simulink model "SignalShapingTest"  (R2024b)
settings: Solver=VariableStepAuto  StartTime=0.0  StopTime=5  RelTol=1e-3
values from neighbouring files (symbols this model uses):
  CanaryAmplitude = 0.25    [ConfigData.sldd]
  CanaryCarrierFrequency = 20000.0    [ConfigData.sldd]
  CanaryDataRate = 100.0    [ConfigData.sldd]
  SampleRate = 48000.0    [ConfigData.sldd]
  WalshCodeIndex = 9.0 3.0    [ConfigData.sldd]
undefined symbols (not defined in the file or in its folder): magnitude
libraries: dspfdesign x5, simulink x3, commseqgen3 x3, commfilt2 x2, dspsigops x2
settings Model: DataDictionary=ConfigData.sldd  Creator=calum  LastModifiedBy=calum

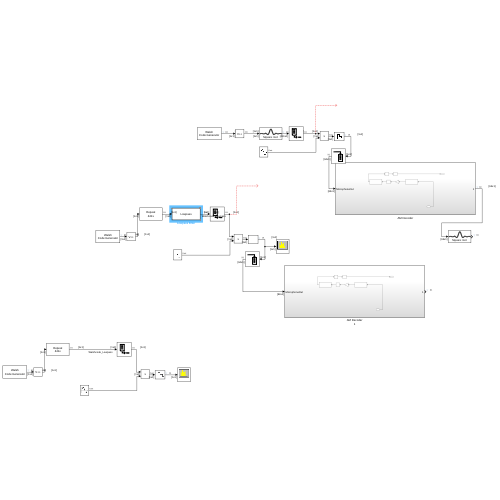
[thumbnail: Simulink's stored preview of the top-level diagram]
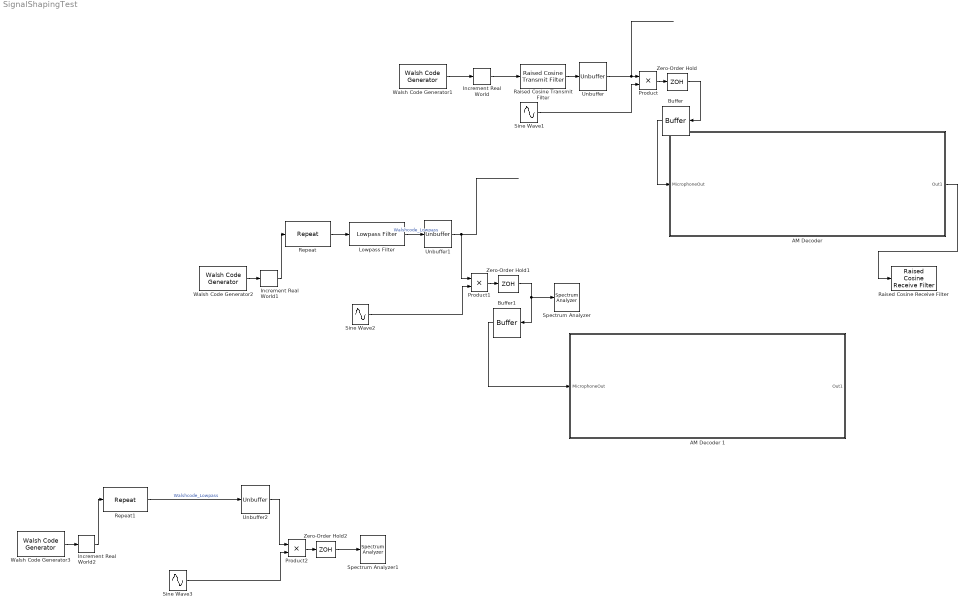
== system SignalShapingTest ==
  "AM Decoder " : Subsystem  Latency=2
  AM Decoder 1 : Subsystem  Latency=2
  Buffer : Buffer  OutputFrames=off
  Buffer1 : Buffer  OutputFrames=off
  Increment Real World : simulink/Additional Math & Discrete/Additional Math: Increment - Decrement/Increment Real World
  Increment Real World1 : simulink/Additional Math & Discrete/Additional Math: Increment - Decrement/Increment Real World
  Increment Real World2 : simulink/Additional Math & Discrete/Additional Math: Increment - Decrement/Increment Real World
  Lowpass Filter : dspfdesign/Lowpass Filter  FilterType=FIR  DesignForMinimumOrder=on  FilterOrder=50  PassbandFrequency=CanaryDataRate  StopbandFrequency=CanaryDataRate*10  PassbandRipple=0.5  StopbandAttenuation=80  SampleRateMode=Specify on dialog  SampleRate=SampleRate  SimulateUsing=Interpreted execution  roundingMode=Floor  coeffsDataTypeStr=fixdt(1,16)
  Product : Product
  Product1 : Product
  Product2 : Product
  Raised Cosine Receive Filter : commfilt2/Raised Cosine Receive Filter  filtType=Square root  R=0.2  filtSpan=2  N=SampleRate/CanaryDataRate  downFactor=1  downOffset=0  filterGain=1  InputProcessing=Columns as channels (frame based)  RateOptions=Allow multirate processing  framing=Mute  checkCoeff=off  variableName=rcRxFilt  currentFiltSpan=10  D=5  inputOffset=0  sampMode=Mute  saveAsFlag=0  rateMode=Downsampling  checkGain=Normalized  launchFVT=on  roundingMode=Floor  overflowMode=off  coeffDataTypeStr=Inherit: Same word length as input  coeffMin=[]  coeffMax=[]  coeffLastDataTypeStr=Inherit: Same word length as input  accumDataTypeStr=Inherit: Same as product output  accumLastDataTypeStr=Inherit: Same as product output  outputDataTypeStr=Inherit: Same as accumulator  outputMin=[]  outputMax=[]  outputLastDataTypeStr=Inherit: Same as accumulator
      settings: LibrarySourceBlock=|
      | commhdlfilt/Raised Cosine
      | Receive Filter
  Raised Cosine Transmit Filter : commfilt2/Raised Cosine Transmit Filter  filtType=Square root  R=0.2  filtSpan=2  N=SampleRate/CanaryDataRate  filterGain=0.5  InputProcessing=Columns as channels (frame based)  RateOptions=Enforce single-rate processing  framing=Mute  checkCoeff=off  variableName=rcTxFilt  checkGain=Normalized  sampMode=Mute  saveAsFlag=0  currentFiltSpan=10  D=(10)/2  launchFVT=on  roundingMode=Floor  overflowMode=off  coeffDataTypeStr=Inherit: Same word length as input  coeffMin=[]  coeffMax=[]  coeffLastDataTypeStr=Inherit: Same word length as input  outputDataTypeStr=Inherit: Same as accumulator  outputMin=[]  outputMax=[]  outputLastDataTypeStr=Inherit: Same as accumulator
  Repeat : dspsigops/Repeat  FactorSource=Dialog parameter  N=SampleRate/CanaryDataRate  Nmax=16  InputProcessing=Columns as channels (frame based)  RateOptions=Allow multirate processing  ic=0  mode=Unused parameter value
      settings: LibrarySourceBlock=commsequence2/Repeat
  Repeat1 : dspsigops/Repeat  FactorSource=Dialog parameter  N=SampleRate/CanaryDataRate  Nmax=16  InputProcessing=Columns as channels (frame based)  RateOptions=Allow multirate processing  ic=0  mode=Unused parameter value
      settings: LibrarySourceBlock=commsequence2/Repeat
  Sine Wave1 : Sin  Amplitude=CanaryAmplitude  Frequency=2*pi*CanaryCarrierFrequency  SampleTime=0
  Sine Wave2 : Sin  Amplitude=CanaryAmplitude  Frequency=2*pi*CanaryCarrierFrequency  SampleTime=0
  Sine Wave3 : Sin  Amplitude=CanaryAmplitude  Frequency=2*pi*CanaryCarrierFrequency  SampleTime=0
  Spectrum Analyzer : SpectrumAnalyzer  WindowPosition=[163.000000,325.000000,939.000000,500.000000,]  Visible=on  ScopeFrameLocation=window  SampleRate=44.1e3  PlotAsTwoSidedSpectrum=off  FrequencyScale=Log  WindowInvariantSamplesPerUpdate=on  FrequencySpan=Start and stop frequencies  StartFrequency=20  StopFrequency=20e3  YLimits=[-90.91644673,38.27949528]  ShowForgettingFactor=on
  Spectrum Analyzer1 : SpectrumAnalyzer  WindowPosition=[1083.000000,318.000000,800.000000,500.000000,]  Visible=on  ScopeFrameLocation=window  SampleRate=44.1e3  PlotAsTwoSidedSpectrum=off  FrequencyScale=Log  WindowInvariantSamplesPerUpdate=on  FrequencySpan=Start and stop frequencies  StartFrequency=20  StopFrequency=20e3  YLimits=[-86.06986587,38.40588463]
  Unbuffer : Unbuffer
  Unbuffer1 : Unbuffer
  Unbuffer2 : Unbuffer
  Walsh Code Generator1 : commseqgen3/Walsh Code Generator  Length=16  Index=WalshCodeIndex(2)  SampleTime=1/CanaryDataRate  SamplesPerFrame=1  OutputDataType=double  SimulateUsing=Code generation
  Walsh Code Generator2 : commseqgen3/Walsh Code Generator  Length=16  Index=WalshCodeIndex(2)  SampleTime=1/CanaryDataRate  SamplesPerFrame=1  OutputDataType=double  SimulateUsing=Code generation
  Walsh Code Generator3 : commseqgen3/Walsh Code Generator  Length=16  Index=WalshCodeIndex(2)  SampleTime=1/CanaryDataRate  SamplesPerFrame=1  OutputDataType=double  SimulateUsing=Code generation
  Zero-Order Hold : ZeroOrderHold  SampleTime=1/SampleRate
  Zero-Order Hold1 : ZeroOrderHold  SampleTime=1/SampleRate
  Zero-Order Hold2 : ZeroOrderHold  SampleTime=1/SampleRate
  wires:
  Walsh Code Generator1/1 -> Increment Real World/1
  Sine Wave1/1 -> Product/2
  Product/1 -> Zero-Order Hold/1
  Raised Cosine Transmit Filter/1 -> Unbuffer/1
  Increment Real World/1 -> Raised Cosine Transmit Filter/1
  Zero-Order Hold/1 -> Buffer/1
  "AM Decoder "/1(Out1) -> Raised Cosine Receive Filter/1
  Unbuffer/1 -> Product/1
  Buffer/1 -> "AM Decoder "/1(MicrophoneOut)
  Buffer1/1 -> AM Decoder 1/1(MicrophoneOut)
  Walsh Code Generator2/1 -> Increment Real World1/1
  Unbuffer1/1 -> Product1/1
  Zero-Order Hold1/1 -> Spectrum Analyzer/1, Buffer1/1
  Increment Real World1/1 -> Repeat/1
  Lowpass Filter/1 -> Unbuffer1/1  "Walshcode_Lowpass"
  Product1/1 -> Zero-Order Hold1/1
  Sine Wave2/1 -> Product1/2
  Repeat/1 -> Lowpass Filter/1
  Increment Real World2/1 -> Repeat1/1
  Walsh Code Generator3/1 -> Increment Real World2/1
  Product2/1 -> Zero-Order Hold2/1
  Unbuffer2/1 -> Product2/1
  Sine Wave3/1 -> Product2/2
  Repeat1/1 -> Unbuffer2/1  "Walshcode_Lowpass"
  Zero-Order Hold2/1 -> Spectrum Analyzer1/1

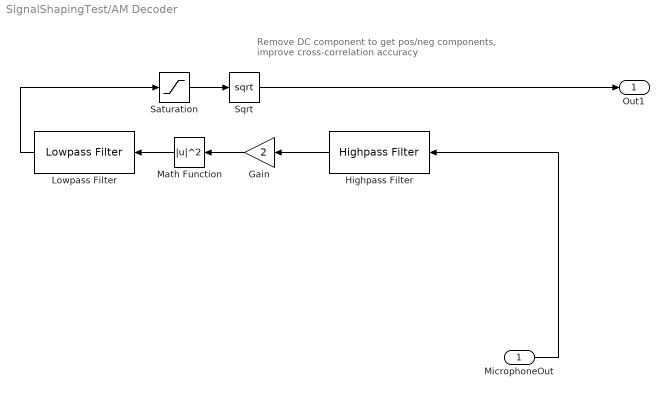
== system SignalShapingTest/AM Decoder  ==
  note: Remove DC component to get pos/neg components,
      | improve cross-correlation accuracy
  MicrophoneOut : Inport
  Gain : Gain  Gain=2
  Highpass Filter : dspfdesign/Highpass Filter  FilterType=FIR  DesignForMinimumOrder=on  FilterOrder=50  StopbandFrequency=CanaryCarrierFrequency-20*CanaryDataRate  PassbandFrequency=CanaryCarrierFrequency-3*CanaryDataRate  StopbandAttenuation=80  PassbandRipple=2  SampleRateMode=Specify on dialog  SampleRate=SampleRate  SimulateUsing=Code generation  roundingMode=Floor  coeffsDataTypeStr=fixdt(1,16)
  Lowpass Filter : dspfdesign/Lowpass Filter  FilterType=FIR  DesignForMinimumOrder=on  FilterOrder=50  PassbandFrequency=CanaryDataRate*2  StopbandFrequency=CanaryDataRate*20  PassbandRipple=0.1  StopbandAttenuation=80  SampleRateMode=Specify on dialog  SampleRate=44100  SimulateUsing=Code generation  roundingMode=Floor  coeffsDataTypeStr=fixdt(1,16)
  Math Function : Math  Operator=magnitude^2
  Saturation : Saturate  UpperLimit=inf  LowerLimit=0
  Sqrt : Sqrt
  Out1 : Outport
  wires:
  Gain/1 -> Math Function/1
  Highpass Filter/1 -> Gain/1
  Sqrt/1 -> Out1/1
  Math Function/1 -> Lowpass Filter/1
  Saturation/1 -> Sqrt/1
  Lowpass Filter/1 -> Saturation/1
  MicrophoneOut/1 -> Highpass Filter/1

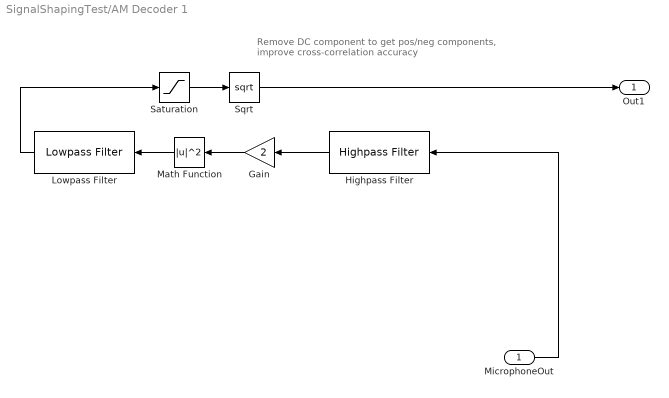
== system SignalShapingTest/AM Decoder 1 ==
  note: Remove DC component to get pos/neg components,
      | improve cross-correlation accuracy
  MicrophoneOut : Inport
  Gain : Gain  Gain=2
  Highpass Filter : dspfdesign/Highpass Filter  FilterType=FIR  DesignForMinimumOrder=on  FilterOrder=50  StopbandFrequency=CanaryCarrierFrequency-20*CanaryDataRate  PassbandFrequency=CanaryCarrierFrequency-3*CanaryDataRate  StopbandAttenuation=80  PassbandRipple=2  SampleRateMode=Specify on dialog  SampleRate=SampleRate  SimulateUsing=Code generation  roundingMode=Floor  coeffsDataTypeStr=fixdt(1,16)
  Lowpass Filter : dspfdesign/Lowpass Filter  FilterType=FIR  DesignForMinimumOrder=on  FilterOrder=50  PassbandFrequency=CanaryDataRate*2  StopbandFrequency=CanaryDataRate*20  PassbandRipple=0.1  StopbandAttenuation=80  SampleRateMode=Specify on dialog  SampleRate=44100  SimulateUsing=Code generation  roundingMode=Floor  coeffsDataTypeStr=fixdt(1,16)
  Math Function : Math  Operator=magnitude^2
  Saturation : Saturate  UpperLimit=inf  LowerLimit=0
  Sqrt : Sqrt
  Out1 : Outport
  wires:
  Gain/1 -> Math Function/1
  Highpass Filter/1 -> Gain/1
  Sqrt/1 -> Out1/1
  Math Function/1 -> Lowpass Filter/1
  Saturation/1 -> Sqrt/1
  Lowpass Filter/1 -> Saturation/1
  MicrophoneOut/1 -> Highpass Filter/1
